simulink model "JenaFox_moodle_ISB"  (R2018b)
settings: Solver=ode23s  StartTime=0.0  StopTime=10  MaxStep=maxStep  RelTol=relTol  AbsTol=absTol
InitFcn:
  | Fox_param;
undefined symbols (not defined in the file): amplifier, c_coupling_hip, c_coupling_knee, c_hs, d_coupling_knee, d_hs, g, hip_i, hip_Jm, hip_k, hip_Mrg, hip_Mrhg, hip_na, hip_Ra, IC_motor_hip_l, IC_motor_hip_r, IC_motor_knee_l, IC_motor_knee_r, IC_phi_hip_l, IC_phi_hip_r, IC_v_motor_hip, IC_v_motor_knee, k_gx, k_gy, knee_i, knee_Jm, knee_k, knee_Mrg, knee_Mrhg, knee_na, knee_Ra, mu_slide, mu_stick, smiData, v_gx_max, v_gy_max, vLimit, X, Y, Z
libraries: sm_lib x38, nesl_utility x26, simulink x16, simulink_extras x8
(part 3 of 3)

== matlab function JenaFox_moodle_ISB/joint voltage calculation ==
  data: U output; phi input; v_phi input; GC input
function U = rb_control(phi,v_phi,GC)%, v_COM)

% calculates the motor torques for the runbot model (method described in Geng 2009 IEEE Trans. Mech.)
% the following indices stand for joint:
% 1 - right hip     3 - right knee
% 2 - left hip      4 - left knee


U=zeros(4,1);
phi_eq=zeros(4,1);

%% define constants

alpha=10;    %gain for equilibrium point calculation in hip joint
bbeta=0.03;  %gain for joint stiffness calculation
gamma=0.001;%base level stiffness
deltah=0.8;   %damping coefficient hip
deltak=0.07; %damping coefficient knee
phi0=-5;    %offset angle [deg]

%a_ext=phi0+2;


%% define motor neuron activity

M_eh=400;      %extensor neuron hip
M_fh=350;      %flexor neuron hip

% scale torques
ht_f=200;      %hip torque in flight
ht_s=250;       %hip torque in stance
kt_s=60;         %knee torque in stance
kt_f=800;    %knee torque in flight

%% calculate torques
K=bbeta*(M_eh+M_fh+gamma);   %21
switch GC
    case 1
        %single support left
        %right leg
        phi_eq(1)=phi0-alpha*(M_eh-M_fh)/K;         %right hip (AEA)
        U(1)=K*(phi_eq(1)-phi(1))-deltah*v_phi(1);
        if phi(1)>phi_eq(1)-1
            U(3)=K*(-90-phi(3))-deltak*v_phi(3);         %right knee bends
        else
            U(3)=K*(2-phi(3))-deltak*v_phi(3);         %right knee stays extended
        end
        %left leg
        phi_eq(2)=phi0+alpha*(M_eh-M_fh)/K;              %left hip (PEA)
        U(2)=K*(phi_eq(2)-phi(2))-deltah*v_phi(2);
        U(4)=K*(2-phi(4))-deltak*v_phi(4);          %left knee extends/stays extended
        % scale torques
        U(1)=U(1)/ht_f;
        U(3)=U(3)/kt_f;
        U(2)=U(2)/ht_s;
        U(4)=U(4)/kt_s;
    case 2
        %double support after touch down right
        %right leg
        phi_eq(1)=phi0+alpha*(M_eh-M_fh)/K;         %right hip(PEA)
        U(1)=K*(phi_eq(1)-phi(1))-deltah*v_phi(1);
        U(3)=K*(2-phi(3))-deltak*v_phi(3);       %right knee extends
        %left leg
        phi_eq(2)=phi0-alpha*(M_eh-M_fh)/K;          %left hip (AEA)
        U(2)=K*(phi_eq(2)-phi(2))-deltah*v_phi(2);
        if phi_eq(2)>phi(2)
            U(4)=K*(2-phi(4))-deltak*v_phi(4);           %left knee stays extended
        else
            U(4)=K*(-90-phi(4))-deltak*v_phi(4);           %left knee starts to flex
        end
        U(1)=U(1)/ht_s;
        U(3)=U(3)/kt_s;
        U(2)=U(2)/ht_s;
        U(4)=U(4)/kt_s;
    case 3
        %single support right leg
        %right leg
        phi_eq(1)=phi0+alpha*(M_eh-M_fh)/K;              %right hip (PEA)
        U(1)=K*(phi_eq(1)-phi(1))-deltah*v_phi(1);
        U(3)=K*(2-phi(3))-deltak*v_phi(3);          %right knee extends/stays extended
        %left leg
        phi_eq(2)=phi0-alpha*(M_eh-M_fh)/K;         %left hip (AEA)
        U(2)=K*(phi_eq(2)-phi(2))-deltah*v_phi(2);
        if phi(2)>phi_eq(2)-1
            U(4)=K*(-90-phi(4))-deltak*v_phi(4);         %left knee bends
        else
            U(4)=K*(2-phi(4))-deltak*v_phi(4);         %left knee stays extended
        end
        U(1)=U(1)/ht_s;
        U(3)=U(3)/kt_s;
        U(2)=U(2)/ht_f;
        U(4)=U(4)/kt_f;
    case 4
        %double support after touch down left
        %right leg
        phi_eq(1)=phi0-alpha*(M_eh-M_fh)/K;          %right hip (AEA)
        U(1)=K*(phi_eq(1)-phi(1))-deltah*v_phi(1);
        if phi_eq(1)>phi(1)
            U(3)=K*(2-phi(3))-deltak*v_phi(3);           %right knee stays extended
        else
            U(3)=K*(-90-phi(3))-deltak*v_phi(3);           %right knee starts to flex
        end
        %left leg
        phi_eq(2)=phi0+alpha*(M_eh-M_fh)/K;         %left hip(AEA)
        U(2)=K*(phi_eq(2)-phi(2))-deltah*v_phi(2);
        U(4)=K*(2-phi(4))-deltak*v_phi(4);       %left knee extends
        U(1)=U(1)/ht_s;
        U(3)=U(3)/kt_s;
        U(2)=U(2)/ht_s;
        U(4)=U(4)/kt_s;
end
